simulink model "change_car"  (Simulink 8.8)
settings: Solver=FixedStepDiscrete  StartTime=0.0  StopTime=30  FixedStep=0.001  RelTol=1e-3
undefined symbols (not defined in the file or in its folder): plecs
libraries: Solver_SF x2, simulink x2
settings Model: Creator=STU  LastModifiedBy=STU
settings DataIOCC: LimitDataPoints=off  SaveFormat=Dataset  SignalLoggingSaveFormat=Dataset
settings OptimizationCC: LifeSpan=auto
settings DebuggingCC: UnderspecifiedInitializationDetection=Simplified  MergeDetectMultiDrivingBlocksExec=error  FcnCallInpInsideContextMsg=error  StateNameClashWarn=none  SFUnexpectedBacktrackingDiag=error  SFNoUnconditionalDefaultTransitionDiag=error  SFExecutionAtInitializationDiag=warning
settings HardwareCC: ProdBitPerPointer=64  ProdBitPerSizeT=64  ProdBitPerPtrDiffT=64  ProdLargestAtomicFloat=Float  ProdIntDivRoundTo=Zero  ProdEndianess=LittleEndian  ProdWordSize=64  ProdHWDeviceType=Intel->x86-64 (Windows64)
settings ModelReferenceCC: PropagateSignalLabelsOutOfModel=on
settings GRTTargetCC: TargetLangStandard=C99 (ISO)  GeneratePreprocessorConditionals=Use local settings  CombineOutputUpdateFcns=on  GRTInterface=off
settings ConfigComp: CovMetricSettings=dwe  CovHtmlReporting=off  CovSaveCumulativeToWorkspaceVar=off  CovSaveSingleToWorkspaceVar=off  CovExternalEMLEnable=on

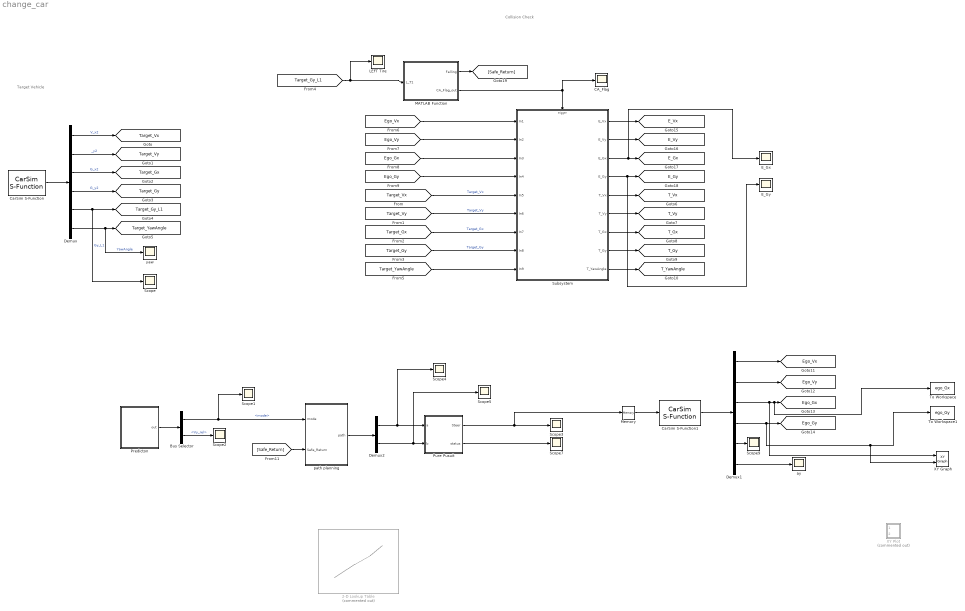
== system change_car ==
  note: Target Vehicle
  note: Collision Check
  2-D Lookup Table : Lookup_n-D  Commented=on  BreakpointsForDimension1=[1:3]  BreakpointsForDimension2=[1:3]  InternalRulePriority=Speed  RndMeth=Simplest  InputSameDT=on
  Bus Selector : BusSelector  OutputSignals=mode,Vy_rel
  CA_Flag : Scope
  CarSim S-Function : Solver_SF/CarSim S-Function  Priority=1  VehicleCode=i_i2  SIMFILE=Second
  CarSim S-Function1 : Solver_SF/CarSim S-Function  Priority=1  VehicleCode=i_i  SIMFILE=First
  Demux : Demux  Outputs=6
  Demux1 : Demux  Outputs=6
  Demux2 : Demux  Outputs=2
  E_Gx : Scope
  E_Gy : Scope
  LEFT Tire : Scope
  MATLAB Function : MATLAB Function  TreatAsAtomicUnit=on
  Memory : Memory
  Predicton : Subsystem
  Pure Pusuit : Subsystem
  Scope{,1..5,7,9} (8 alike) : Scope
  Subsystem : Subsystem
  To Workspace : ToWorkspace  VariableName=ego_Gx  SampleTime=-1
  To Workspace1 : ToWorkspace  VariableName=ego_Gy  SampleTime=-1
  XY Graph : simulink/Sinks/XY Graph  xmin=-1  xmax=1  ymin=-1  ymax=1  st=-1
  XY Plot : Subsystem  Commented=on  LoadFcn=plecs('sl', 317);  InitFcn=plecs('sl', 314);  StartFcn=plecs('sl', 308);  StopFcn=plecs('sl', 309);  mask{Settings=<binary blob, 240 chars, not shown>}
      mask init:
      | plecs('sl', 315);
      settings: CopyFcn=plecs('sl', 318);  DeleteFcn=plecs('sl', 305);  UndoDeleteFcn=plecs('sl', 306);  PreSaveFcn=plecs('sl', 311);  NameChangeFcn=plecs('sl', 310);  DestroyFcn=plecs('sl', 307);  OpenFcn=plecs('sl', 302);  ErrorFcn=plerrorfcn
      mask Display:
      | plot([0.05 0.95 0.95 0.05 0.05], [0.95 0.95 0.05 0.05 0.95])
      | plot(0.5+sin((0:0.2:2)*pi)*0.3, 0.5+sin((0:0.2:2)*pi + pi/4)*0.3);
  ay : Scope
  path planning : Subsystem
  yaw : Scope
  tag scope: E_Gx=global, E_Gy=global, E_Vx=global, E_Vy=global, Ego_Gx=global, Ego_Gy=global, Ego_Vx=global, Ego_Vy=global, T_Gx=global, T_Gy=global, T_Vx=global, T_Vy=global, T_YawAngle=global, Target_Gx=global, Target_Gy=global, Target_Gy_L1=global, Target_Vx=global, Target_Vy=global, Target_YawAngle=global
  wires:
  CarSim S-Function/1 -> Demux/1
  Demux/1 -> [Target_Vx]  "V_x2"
  Demux/2 -> [Target_Vy]  "_y2"
  Demux/3 -> [Target_Gx]  "G_x2"
  Demux/4 -> [Target_Gy]  "G_y2"
  CarSim S-Function1/1 -> Demux1/1
  Demux1/5 -> Scope9/1
  Demux/5 -> Scope/1, [Target_Gy_L1]  "Gy_L1"
  Demux/6 -> yaw/1, [Target_YawAngle]  "YawAngle"
  MATLAB Function/2(CA_Flag_out) -> CA_Flag/1, Subsystem/Trigger
  [Target_Gy_L1] -> MATLAB Function/1(L_T1), LEFT Tire/1
  Demux1/4 -> To Workspace1/1, XY Graph/2, [Ego_Gy]
  Demux1/3 -> XY Graph/1, To Workspace/1, [Ego_Gx]
  Demux1/2 -> [Ego_Vy]
  Demux1/1 -> [Ego_Vx]
  [Ego_Vx] -> Subsystem/1(In1)
  [Ego_Vy] -> Subsystem/2(In2)
  [Ego_Gx] -> Subsystem/3(In3)
  [Ego_Gy] -> Subsystem/4(In4)
  [Target_Vx] -> Subsystem/5(In5)  "Target_Vx"
  [Target_Vy] -> Subsystem/6(In6)  "Target_Vy"
  [Target_Gx] -> Subsystem/7(In7)  "Target_Gx"
  [Target_Gy] -> Subsystem/8(In8)  "Target_Gy"
  [Target_YawAngle] -> Subsystem/9(In9)
  Subsystem/5(T_Vx) -> [T_Vx]
  Subsystem/6(T_Vy) -> [T_Vy]
  Subsystem/7(T_Gx) -> [T_Gx]
  Subsystem/8(T_Gy) -> [T_Gy]
  Subsystem/9(T_YawAngle) -> [T_YawAngle]
  Subsystem/1(E_Vx) -> [E_Vx]
  Subsystem/2(E_Vy) -> [E_Vy]
  Subsystem/3(E_Gx) -> E_Gx/1, [E_Gx]
  Subsystem/4(E_Gy) -> E_Gy/1, [E_Gy]
  Predicton/1(out) -> Bus Selector/1
  Bus Selector/2 -> Scope2/1  "<Vy_rel>"
  Bus Selector/1 -> Scope1/1, path planning/1(mode)  "<mode>"
  path planning/1(path) -> Demux2/1
  Demux2/1 -> Pure Pusuit/1(a), Scope4/1
  Demux2/2 -> Scope5/1, Pure Pusuit/2(b)
  Pure Pusuit/2(status) -> Scope7/1
  MATLAB Function/1(Falling) -> [Safe_Return]
  [Safe_Return] -> path planning/2(Safe_Return)
  Demux1/6 -> ay/1
  Memory/1 -> CarSim S-Function1/1
  Pure Pusuit/1(Steer) -> Scope3/1, Memory/1

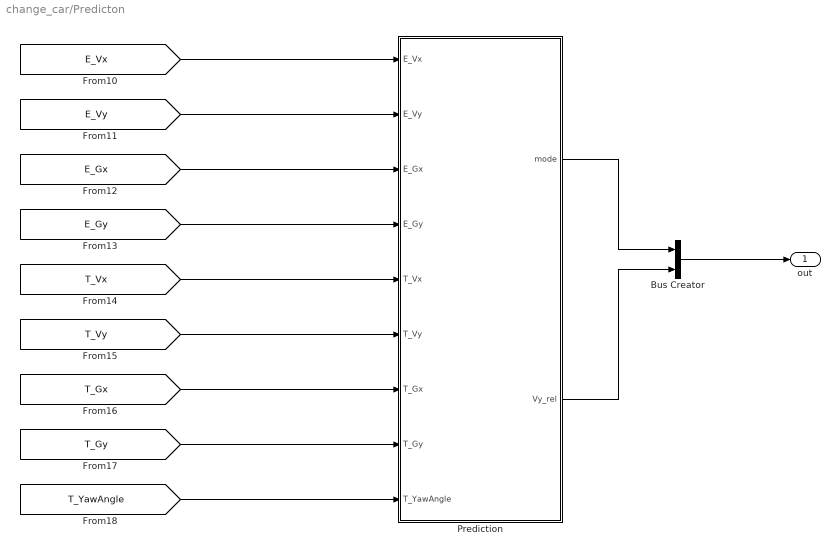
== system change_car/Predicton ==
  Bus Creator : BusCreator  Inputs=2
  Prediction : MATLAB Function  TreatAsAtomicUnit=on
  out : Outport
  wires:
  [E_Vx] -> Prediction/1(E_Vx)
  [E_Vy] -> Prediction/2(E_Vy)
  [E_Gx] -> Prediction/3(E_Gx)
  [E_Gy] -> Prediction/4(E_Gy)
  [T_Vx] -> Prediction/5(T_Vx)
  [T_Vy] -> Prediction/6(T_Vy)
  [T_Gx] -> Prediction/7(T_Gx)
  [T_Gy] -> Prediction/8(T_Gy)
  [T_YawAngle] -> Prediction/9(T_YawAngle)
  Prediction/1(mode) -> Bus Creator/1
  Prediction/2(Vy_rel) -> Bus Creator/2
  Bus Creator/1 -> out/1

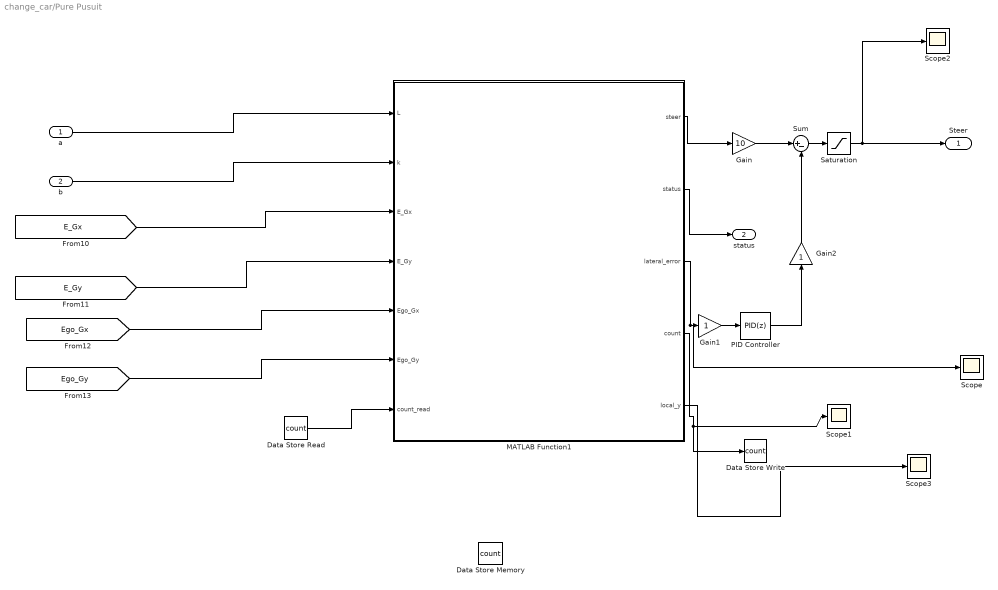
== system change_car/Pure Pusuit ==
  a : Inport
  b : Inport  Port=2
  Data Store Memory : DataStoreMemory  DataStoreName=count  ReadBeforeWriteMsg=warning  WriteAfterWriteMsg=warning  WriteAfterReadMsg=warning  ShowAdditionalParam=off  OutDataTypeStr=double
  Data Store Read : DataStoreRead  DataStoreName=count  DataStoreElements=count
  Data Store Write : DataStoreWrite  DataStoreName=count  DataStoreElements=count
  Gain : Gain  Gain=10
  Gain1 : Gain
  Gain2 : Gain
  MATLAB Function1 : MATLAB Function  TreatAsAtomicUnit=on
  PID Controller : simulink/Continuous/PID Controller  Controller=PID  TimeDomain=Discrete-time  SampleTime=-1  IntegratorMethod=Forward Euler  FilterMethod=Forward Euler  Form=Parallel  UseFilter=on  ControllerParametersSource=internal  P=1  I=0.1  D=40  N=100  InitialConditionSource=internal  InitialConditionForIntegrator=0  InitialConditionForFilter=0  ExternalReset=none  LimitOutput=off  UpperSaturationLimit=inf  LowerSaturationLimit=-inf  LinearizeAsGain=on  AntiWindupMode=none  Kb=1  TrackingMode=off  Kt=1  PParamMin=[]  PParamMax=[]  IParamMin=[]  IParamMax=[]  DParamMin=[]  DParamMax=[]  NParamMin=[]  NParamMax=[]  KbParamMin=[]  KbParamMax=[]  KtParamMin=[]  KtParamMax=[]  POutMin=[]  POutMax=[]  IOutMin=[]  IOutMax=[]  DOutMin=[]  DOutMax=[]  NOutMin=[]  NOutMax=[]  KbOutMin=[]  KbOutMax=[]  KtOutMin=[]  KtOutMax=[]  IntegratorOutMin=[]  IntegratorOutMax=[]  FilterOutMin=[]  FilterOutMax=[]  SumOutMin=[]  SumOutMax=[]  SumI1OutMin=[]  SumI1OutMax=[]  SumI2OutMin=[]  SumI2OutMax=[]  SumI3OutMin=[]  SumI3OutMax=[]  SumDOutMin=[]  SumDOutMax=[]  SaturationOutMin=[]  SaturationOutMax=[]  IntegratorContinuousStateAttributes=''  IntegratorStateMustResolveToSignalObject=off  IntegratorRTWStateStorageClass=Auto  FilterContinuousStateAttributes=''  FilterStateMustResolveToSignalObject=off  FilterRTWStateStorageClass=Auto  DifferentiatorICPrevScaledInput=0  DifferentiatorOutMin=[]  DifferentiatorOutMax=[]
  Saturation : Saturate  UpperLimit=30  LowerLimit=-30
  Scope{,1..3} (4 alike) : Scope
  Sum : Sum  Inputs=|+-
  Steer : Outport
  status : Outport  Port=2
  wires:
  a/1 -> MATLAB Function1/1(L)
  [Ego_Gy] -> MATLAB Function1/6(Ego_Gy)
  [E_Gx] -> MATLAB Function1/3(E_Gx)
  [E_Gy] -> MATLAB Function1/4(E_Gy)
  [Ego_Gx] -> MATLAB Function1/5(Ego_Gx)
  b/1 -> MATLAB Function1/2(k)
  MATLAB Function1/2(status) -> status/1
  MATLAB Function1/3(lateral_error) -> Gain1/1, Scope/1
  PID Controller/1 -> Gain2/1
  Sum/1 -> Saturation/1
  Gain/1 -> Sum/1
  MATLAB Function1/1(steer) -> Gain/1
  Gain1/1 -> PID Controller/1
  Data Store Read/1 -> MATLAB Function1/7(count_read)
  MATLAB Function1/4(count) -> Data Store Write/1, Scope1/1
  Gain2/1 -> Sum/2
  MATLAB Function1/5(local_y) -> Scope3/1
  Saturation/1 -> Steer/1, Scope2/1

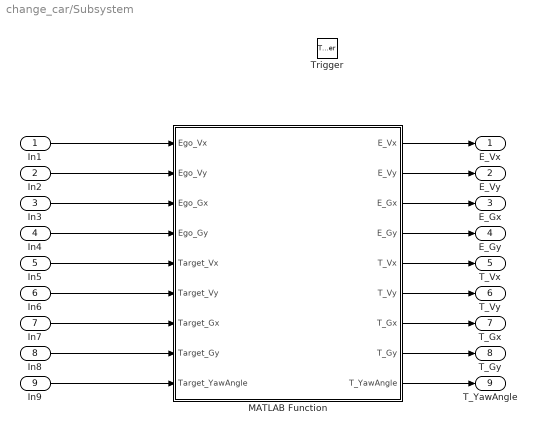
== system change_car/Subsystem ==
  In1 : Inport
  In2 : Inport  Port=2
  In3 : Inport  Port=3
  In4 : Inport  Port=4
  In5 : Inport  Port=5
  In6 : Inport  Port=6
  In7 : Inport  Port=7
  In8 : Inport  Port=8
  In9 : Inport  Port=9
  Trigger : TriggerPort  VariantControl=Variant  PortDimensions=1
  MATLAB Function : MATLAB Function  TreatAsAtomicUnit=on
  E_Vx : Outport
  E_Vy : Outport  Port=2
  E_Gx : Outport  Port=3
  E_Gy : Outport  Port=4
  T_Vx : Outport  Port=5
  T_Vy : Outport  Port=6
  T_Gx : Outport  Port=7
  T_Gy : Outport  Port=8
  T_YawAngle : Outport  Port=9
  wires:
  In1/1 -> MATLAB Function/1(Ego_Vx)
  In2/1 -> MATLAB Function/2(Ego_Vy)
  In3/1 -> MATLAB Function/3(Ego_Gx)
  In4/1 -> MATLAB Function/4(Ego_Gy)
  In5/1 -> MATLAB Function/5(Target_Vx)
  In6/1 -> MATLAB Function/6(Target_Vy)
  In7/1 -> MATLAB Function/7(Target_Gx)
  In8/1 -> MATLAB Function/8(Target_Gy)
  In9/1 -> MATLAB Function/9(Target_YawAngle)
  MATLAB Function/1(E_Vx) -> E_Vx/1
  MATLAB Function/2(E_Vy) -> E_Vy/1
  MATLAB Function/3(E_Gx) -> E_Gx/1
  MATLAB Function/4(E_Gy) -> E_Gy/1
  MATLAB Function/5(T_Vx) -> T_Vx/1
  MATLAB Function/6(T_Vy) -> T_Vy/1
  MATLAB Function/7(T_Gx) -> T_Gx/1
  MATLAB Function/8(T_Gy) -> T_Gy/1
  MATLAB Function/9(T_YawAngle) -> T_YawAngle/1

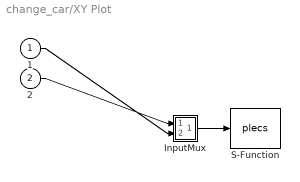
== system change_car/XY Plot ==
  1 : Inport
  2 : Inport  Port=2
  " InputMux " : Subsystem
      mask Display: disp('Mux')
  " S-Function " : S-Function  FunctionName=plecs  SFunctionDeploymentMode=off  EnableBusSupport=off
  wires:
  2/1 -> " InputMux "/1(In1)
  1/1 -> " InputMux "/2(In2)
  " InputMux "/1(Out) -> " S-Function "/1

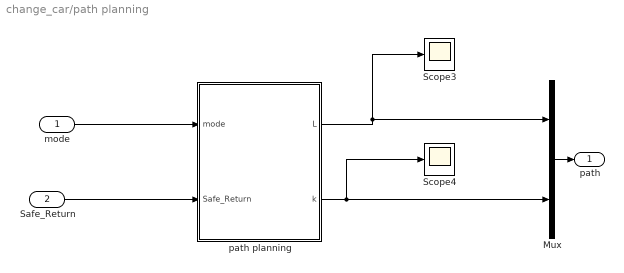
== system change_car/path planning ==
  mode : Inport
  Safe_Return : Inport  Port=2
  Mux : Mux  Inputs=2
  Scope3 : Scope
  Scope4 : Scope
  path planning : MATLAB Function  TreatAsAtomicUnit=on
  path : Outport
  wires:
  path planning/1(L) -> Scope3/1, Mux/1
  path planning/2(k) -> Scope4/1, Mux/2
  Mux/1 -> path/1
  mode/1 -> path planning/1(mode)
  Safe_Return/1 -> path planning/2(Safe_Return)

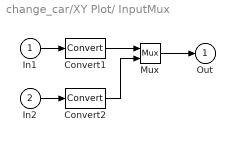
== system change_car/XY Plot/ InputMux  ==
  In1 : Inport
  In2 : Inport  Port=2
  Convert1 : DataTypeConversion  SaturateOnIntegerOverflow=on  RndMeth=Zero
  Convert2 : DataTypeConversion  SaturateOnIntegerOverflow=on  RndMeth=Zero
  Mux : Mux  Inputs=2
  Out : Outport
  wires:
  Convert2/1 -> Mux/2
  In2/1 -> Convert2/1
  Convert1/1 -> Mux/1
  In1/1 -> Convert1/1
  Mux/1 -> Out/1

== matlab function MATLAB Function ==
  data: L_T1 input double; Falling output double; CA_Flag_out output double
function [Falling,CA_Flag_out] = fcn(L_T1)


persistent Fal_Counter CA_Flag_old

if isempty(Fal_Counter)
    Fal_Counter = 0;
    CA_Flag_old = 0;
end

%% Observe 
if L_T1 >= -1.8
    CA_Flag = 1;
else
    CA_Flag = 0;
end

%% Flag Counter
if CA_Flag_old - CA_Flag  == 1
    Fal_Counter = Fal_Counter + 1;
end
Falling = Fal_Counter;

CA_Flag_old = CA_Flag;
CA_Flag_out = CA_Flag_old;

== matlab function Subsystem/MATLAB Function ==
  data: Ego_Vx input double; Ego_Vy input double; Ego_Gx input double; Ego_Gy input double; E_Vx output double; E_Vy output double; E_Gx output double; E_Gy output double; Target_Vx input double; T_Vx output double; Target_Vy input double; Target_Gx input double; Target_Gy input double; T_Vy output double; T_Gx output double; T_Gy output double; Target_YawAngle input double; T_YawAngle output double
function [E_Vx,E_Vy,E_Gx,E_Gy,T_Vx,T_Vy,T_Gx,T_Gy,T_YawAngle] = fcn(Ego_Vx,Ego_Vy,Ego_Gx,Ego_Gy,Target_Vx,Target_Vy,Target_Gx,Target_Gy,Target_YawAngle)
E_Vx = Ego_Vx;
E_Vy = Ego_Vy;
E_Gx = Ego_Gx;
E_Gy = Ego_Gy;
T_Vx = Target_Vx;
T_Vy = Target_Vy;
T_Gx = Target_Gx;
T_Gy = Target_Gy;
T_YawAngle = Target_YawAngle;

== matlab function Predicton/Prediction ==
  data: E_Vx input double; mode output double; E_Vy input double; E_Gx input double; E_Gy input double; T_Vx input double; T_Vy input double; T_Gx input double; T_Gy input double; T_YawAngle input double; Vy_rel output double
function [mode, Vy_rel] = prediction(E_Vx,E_Vy,E_Gx,E_Gy,T_Vx,T_Vy,T_Gx,T_Gy,T_YawAngle)
     if T_Gx == 0
        mode = 0;
        Vy_rel =0;
     else
        predict_time =1;
        T_Yawrad = T_YawAngle * pi/180;
        Global_T_Vx = T_Vx*cos(T_Yawrad) - T_Vy*sin(T_Yawrad);
        Global_T_Vy = T_Vx*sin(T_Yawrad) + T_Vy*cos(T_Yawrad);
        Vx_rel = (Global_T_Vx - E_Vx) / 3.6; %%km/h - > m/s
        Vy_rel = (Global_T_Vy - E_Vy) / 3.6; %%km/h - > m/s
        X_rel = T_Gx - E_Gx;
        Y_rel = T_Gy - E_Gy;

        X_predict = X_rel + Vx_rel * predict_time;
        Y_predict = Y_rel + Vy_rel * predict_time;

        if X_predict >= 20
            mode = 0;
        else
            if Y_predict < -1.8
                mode = 0;               %%keeping current lane
            elseif Y_predict < -0.9
                mode = 1;               %%in-lane chagne 
            else
                mode = 2;
            end
        end
     end

== matlab function path planning/path planning ==
  data: mode input double; L output double; k output double; Safe_Return input double
function [L,k] = path_planning(mode,Safe_Return)



if mode == 1 % Inlane
    if Safe_Return == 2 
        
        L= -1.8;
        k = 0.5;
    else
        L= 1.8;
        k = 0.5;
        
    end
elseif mode == 2 % Lane Change
    L= 7.2;
    k = 1;
else
    L=0;
    k = 0;
end



end

== matlab function Pure Pusuit/MATLAB Function1 ==
  data: L input double; steer output double; k input double; E_Gx input double; E_Gy input double; Ego_Gx input double; Ego_Gy input double; status output double; lateral_error output double; count_read input double; count output double; local_y output double
function [steer,status,lateral_error,count,local_y] = fcn(L,k,E_Gx, E_Gy, Ego_Gx,Ego_Gy,count_read)
    L_v = 2.91;
    k_p = 0.3;
    if count_read == 1
        count = 1;
    else
        count = 0;
    end
    
    if L == 0 && k == 0
        steer = 0;
        status = 0; %%not predicted yet
        lateral_error = 0;
        count = 0;
        local_y = 0;
    else
        local_x = Ego_Gx - E_Gx;
        local_y = Ego_Gy - E_Gy;
        if local_y == L-1
            count =1;
        end
        if count_read == 1
            count = 1;
            k_p = 1;
        end

        l_d = k_p * 90/3.6;

        
 
    %%(x - local_x)^2 + (L/(1+exp(-k*x)) -0.5 - local_y)^2 == (l_d)^2;
    % y = L/(1+e^(-k*x)) -0.5;
%         fun = @(x) (x - local_x)^2 + (L/(1+exp(-k*x)) -0.5 - local_y)^2 - (l_d)^2;
%         h = fzero(fun, [local_x-l_d local_x+2*l_d]);
%         h= h(imag(h)==0);
%         if isempty(h) == 1
%             steer = 0;
%             status = 2; %%no root
%             len = 0;
%         else
       x_pos = local_x + l_d;
       lateral_error =local_y - L / (1+exp(-k*local_x)) + L/2;
       y_pos = L/(1+exp(-k*x_pos)) - L/2;
       e_ld = y_pos - local_y;
       l_d = sqrt((x_pos - local_x)^2 + (y_pos - local_y)^2);
       sin_alpha = e_ld / l_d;
       steer = atan(2*L_v*sin_alpha/l_d)/pi*180;
       status = 1 ; %% predicted
%         end
    end


end
